simulink model "optimum_control"  (R2016a)
settings: Solver=FixedStepAuto  StartTime=0.0  StopTime=30  FixedStep=0.01  RelTol=1e-3
values from neighbouring files (symbols this model uses):
  d0 = 0.5    [optimum_Para.m]
  Kd = 3    [optimum_Para.m]
  Kp = 3    [optimum_Para.m]
  L = 1.06    [optimum_Para.m]
  theta0 = 0    [optimum_Para.m]
  v = 1.5    [optimum_Para.m]
libraries: simulink x1
settings Model: Creator=tangxiaotao  LastModifiedBy=frank lee

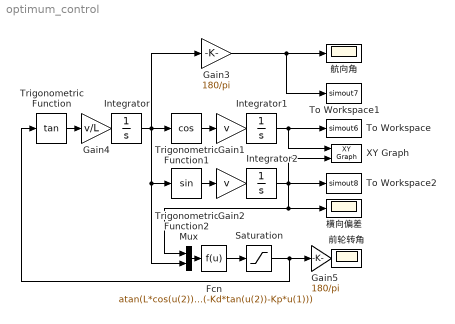
== system optimum_control ==
  Fcn : Fcn  Expr=atan(L*cos(u(2))^3*(-Kd*tan(u(2))-Kp*u(1)))
  Gain1 : Gain  Gain=v
  Gain2 : Gain  Gain=v
  Gain3 : Gain  Gain=180/pi
  Gain4 : Gain  Gain=v/L
  Gain5 : Gain  Gain=180/pi
  Integrator : Integrator  InitialCondition=theta0
  Integrator1 : Integrator
  Integrator2 : Integrator  InitialCondition=d0
  Mux : Mux  Inputs=2
  Saturation : Saturate  UpperLimit=pi/3  LowerLimit=-pi/3
  To Workspace : ToWorkspace  VariableName=simout6  SaveFormat=Timeseries  SampleTime=-1
  To Workspace1 : ToWorkspace  VariableName=simout7  SaveFormat=Timeseries  SampleTime=-1
  To Workspace2 : ToWorkspace  VariableName=simout8  SaveFormat=Timeseries  SampleTime=-1
  Trigonometric Function : Trigonometry  Operator=tan
  Trigonometric Function1 : Trigonometry  Operator=cos
  Trigonometric Function2 : Trigonometry
  XY Graph : simulink/Sinks/XY Graph  xmin=0  xmax=30  ymin=-1  ymax=1  st=-1
  前轮转角 : Scope
  横向偏差 : Scope
  航向角 : Scope
  wires:
  Trigonometric Function/1 -> Gain4/1
  Trigonometric Function1/1 -> Gain1/1
  Trigonometric Function2/1 -> Gain2/1
  Fcn/1 -> Saturation/1
  Integrator/1 -> Mux/2, Trigonometric Function2/1, Gain3/1, Trigonometric Function1/1
  Gain1/1 -> Integrator1/1
  Gain2/1 -> Integrator2/1
  Mux/1 -> Fcn/1
  Gain3/1 -> To Workspace1/1, 航向角/1
  Gain4/1 -> Integrator/1
  Gain5/1 -> 前轮转角/1
  Integrator1/1 -> To Workspace/1, XY Graph/1
  Saturation/1 -> Trigonometric Function/1, Gain5/1
  Integrator2/1 -> Mux/1, 横向偏差/1, XY Graph/2, To Workspace2/1
